simulink model "Q3_simulink"  (R2020b)
settings: Solver=VariableStepAuto  StartTime=0.0  StopTime=800  RelTol=1e-3
settings Model: Creator=User  LastModifiedBy=User

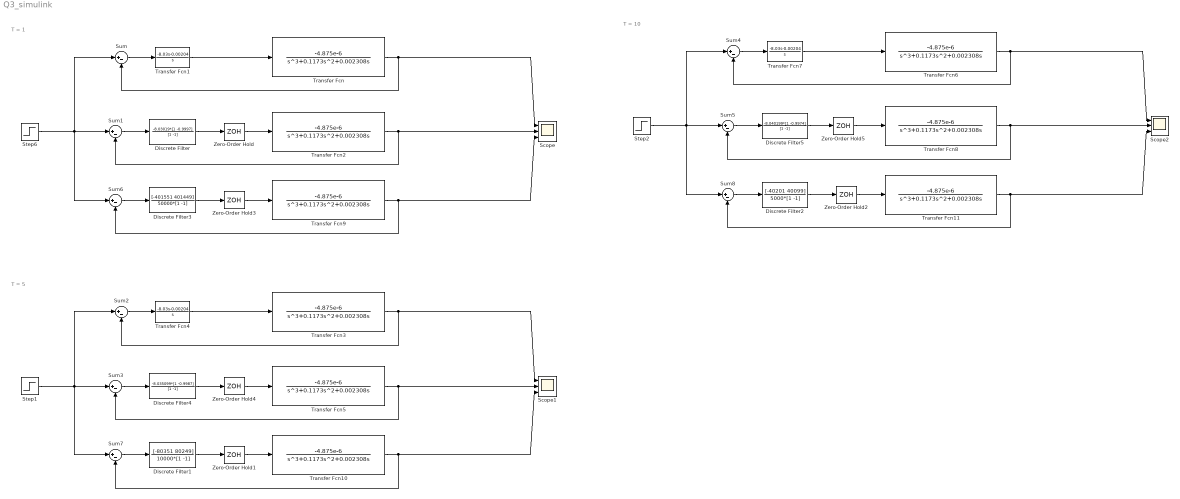
== system Q3_simulink ==
  note: T = 1
  note: T = 5
  note: T = 10
  Discrete Filter : DiscreteFilter  Numerator=-8.03019*[1 -0.9997]  Denominator=[1 -1]  SampleTime=1
  Discrete Filter1 : DiscreteFilter  Numerator=[-80351 80249]  Denominator=10000*[1 -1]  SampleTime=5
  Discrete Filter2 : DiscreteFilter  Numerator=[-40201 40099]  Denominator=5000*[1 -1]  SampleTime=10
  Discrete Filter3 : DiscreteFilter  Numerator=[-401551 401449]  Denominator=50000*[1 -1]  SampleTime=1
  Discrete Filter4 : DiscreteFilter  Numerator=-8.035099*[1 -0.9987]  Denominator=[1 -1]  SampleTime=5
  Discrete Filter5 : DiscreteFilter  Numerator=-8.040199*[1 -0.9974]  Denominator=[1 -1]  SampleTime=10
  Scope : Scope  NumInputPorts=3
  Scope1 : Scope  NumInputPorts=3
  Scope2 : Scope  NumInputPorts=3
  Step1 : Step  Time=0  SampleTime=0
  Step2 : Step  Time=0  SampleTime=0
  Step6 : Step  Time=0  SampleTime=0
  Sum{,1..8} (9 alike) : Sum  Inputs=|+-
  Transfer Fcn{,2..3,5..6,8..11} (9 alike) : TransferFcn  Numerator=[-4.875e-6]  Denominator=[1 0.1173 0.002308 0]
  Transfer Fcn1 : TransferFcn  Numerator=[-8.03 -0.00204]  Denominator=[1 0]
  Transfer Fcn4 : TransferFcn  Numerator=[-8.03 -0.00204]  Denominator=[1 0]
  Transfer Fcn7 : TransferFcn  Numerator=[-8.03 -0.00204]  Denominator=[1 0]
  Zero-Order Hold : ZeroOrderHold
  Zero-Order Hold1 : ZeroOrderHold  SampleTime=5
  Zero-Order Hold2 : ZeroOrderHold  SampleTime=10
  Zero-Order Hold3 : ZeroOrderHold
  Zero-Order Hold4 : ZeroOrderHold  SampleTime=5
  Zero-Order Hold5 : ZeroOrderHold  SampleTime=10
  wires:
  Transfer Fcn1/1 -> Transfer Fcn/1
  Transfer Fcn/1 -> Sum/2, Scope/1
  Sum/1 -> Transfer Fcn1/1
  Zero-Order Hold/1 -> Transfer Fcn2/1
  Discrete Filter/1 -> Zero-Order Hold/1
  Transfer Fcn2/1 -> Scope/2, Sum1/2
  Sum1/1 -> Discrete Filter/1
  Step6/1 -> Sum/1, Sum1/1, Sum6/1
  Sum6/1 -> Discrete Filter3/1
  Transfer Fcn9/1 -> Scope/3, Sum6/2
  Discrete Filter3/1 -> Zero-Order Hold3/1
  Zero-Order Hold3/1 -> Transfer Fcn9/1
  Zero-Order Hold1/1 -> Transfer Fcn10/1
  Discrete Filter1/1 -> Zero-Order Hold1/1
  Transfer Fcn10/1 -> Sum7/2, Scope1/3
  Sum7/1 -> Discrete Filter1/1
  Step1/1 -> Sum7/1, Sum3/1, Sum2/1
  Sum3/1 -> Discrete Filter4/1
  Transfer Fcn5/1 -> Sum3/2, Scope1/2
  Discrete Filter4/1 -> Zero-Order Hold4/1
  Zero-Order Hold4/1 -> Transfer Fcn5/1
  Sum2/1 -> Transfer Fcn4/1
  Transfer Fcn3/1 -> Scope1/1, Sum2/2
  Transfer Fcn4/1 -> Transfer Fcn3/1
  Zero-Order Hold2/1 -> Transfer Fcn11/1
  Discrete Filter2/1 -> Zero-Order Hold2/1
  Transfer Fcn11/1 -> Sum8/2, Scope2/3
  Sum8/1 -> Discrete Filter2/1
  Step2/1 -> Sum8/1, Sum5/1, Sum4/1
  Sum5/1 -> Discrete Filter5/1
  Transfer Fcn8/1 -> Sum5/2, Scope2/2
  Discrete Filter5/1 -> Zero-Order Hold5/1
  Zero-Order Hold5/1 -> Transfer Fcn8/1
  Sum4/1 -> Transfer Fcn7/1
  Transfer Fcn6/1 -> Scope2/1, Sum4/2
  Transfer Fcn7/1 -> Transfer Fcn6/1
